simulink model "fisTreesim"  (R2018a)
settings: Solver=VariableStepAuto  StartTime=0.0  StopTime=10.0  RelTol=1e-3
libraries: fuzblock x3
settings Model: Creator=laksh  LastModifiedBy=laksh

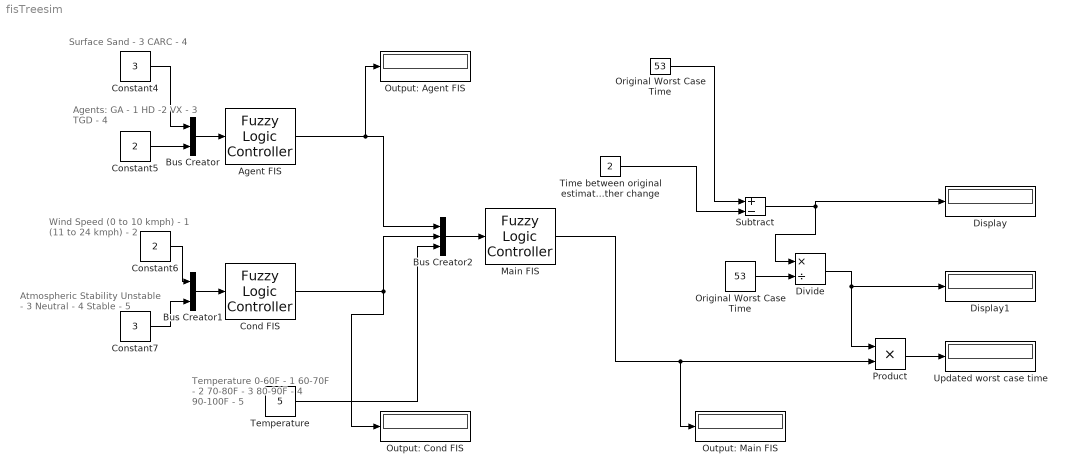
== system fisTreesim ==
  note: Temperature
      | 0-60F - 1
      | 60-70F - 2
      | 70-80F - 3
      | 80-90F - 4
      | 90-100F - 5
  note: Atmospheric Stability
      | Unstable - 3
      | Neutral - 4
      | Stable - 5
  note: Wind Speed
      | (0 to 10 kmph) - 1
      | (11 to 24 kmph) - 2
  note: Surface
      | Sand - 3
      | CARC - 4
  note: Agents:
      | GA - 1
      | HD -2
      | VX - 3
      | TGD - 4
  Agent FIS : fuzblock/Fuzzy Logic  Controller  FIS='AgentFISModel.fis'  OutputSampleNumber=101  DataType=double  FuzzifiedInputs=off  RuleFiringStrengths=off  RuleOutputs=off  AggregatedOutputs=off  SimulateUsing=Interpreted execution  OutOfRangeInputValueMessage=warning  NoRuleFiredMessage=warning  EmptyOutputFuzzySetMessage=warning
  Bus Creator : BusCreator  Inputs=2
  Bus Creator1 : BusCreator  Inputs=2
  Bus Creator2 : BusCreator  Inputs=3
  Cond FIS : fuzblock/Fuzzy Logic  Controller  FIS='condFISModel.fis'  OutputSampleNumber=101  DataType=double  FuzzifiedInputs=off  RuleFiringStrengths=off  RuleOutputs=off  AggregatedOutputs=off  SimulateUsing=Interpreted execution  OutOfRangeInputValueMessage=warning  NoRuleFiredMessage=warning  EmptyOutputFuzzySetMessage=warning
  Constant4 : Constant  Value=3
  Constant5 : Constant  Value=2
  Constant6 : Constant  Value=2
  Constant7 : Constant  Value=3
  Display : Display
  Display1 : Display
  Divide : Product  Inputs=*/
  Main FIS : fuzblock/Fuzzy Logic  Controller  FIS='mainFISModel.fis'  OutputSampleNumber=101  DataType=double  FuzzifiedInputs=off  RuleFiringStrengths=off  RuleOutputs=off  AggregatedOutputs=off  SimulateUsing=Interpreted execution  OutOfRangeInputValueMessage=warning  NoRuleFiredMessage=warning  EmptyOutputFuzzySetMessage=warning
  "Original Worst Case Time " : Constant  Value=53
  Original Worst Case Time : Constant  Value=53
  Output: Agent FIS : Display
  Output: Cond FIS : Display
  Output: Main FIS : Display
  Product : Product
  Subtract : Sum  Inputs=+-
  Temperature : Constant  Value=5
  Time between original estimate and weather change : Constant  Value=2
  Updated worst case time : Display
  wires:
  "Original Worst Case Time "/1 -> Subtract/1
  Time between original estimate and weather change/1 -> Subtract/2
  Subtract/1 -> Display/1, Divide/1
  Original Worst Case Time/1 -> Divide/2
  Divide/1 -> Display1/1, Product/1
  Main FIS/1 -> Output: Main FIS/1, Product/2
  Product/1 -> Updated worst case time/1
  Constant4/1 -> Bus Creator/1
  Constant5/1 -> Bus Creator/2
  Bus Creator/1 -> Agent FIS/1
  Constant6/1 -> Bus Creator1/1
  Constant7/1 -> Bus Creator1/2
  Bus Creator1/1 -> Cond FIS/1
  Agent FIS/1 -> Output: Agent FIS/1, Bus Creator2/1
  Cond FIS/1 -> Output: Cond FIS/1, Bus Creator2/2
  Temperature/1 -> Bus Creator2/3
  Bus Creator2/1 -> Main FIS/1
